simulink model "exp3"  (R2019a)
settings: Solver=FixedStepAuto  StartTime=0.0  StopTime=1e-1  FixedStep=1e-7  RelTol=1e-3
libraries: dsparch4 x1, simulink x1
settings Model: Creator=marco  LastModifiedBy=marco

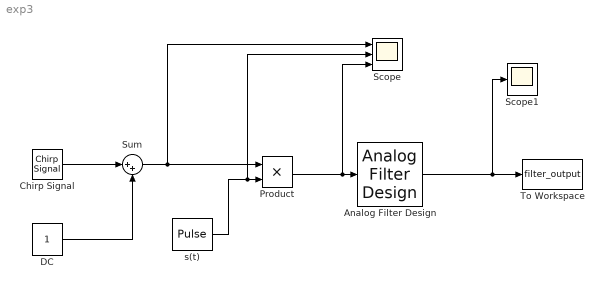
== system exp3 ==
  Analog Filter Design : dsparch4/Analog Filter Design  method=Butterworth  filttype=Bandpass  N=3  Wlo=2*pi*980e3  Whi=2*pi*1020e3  Rp=2  Rs=40
  Chirp Signal : simulink/Sources/Chirp Signal  f1=100  T=0.1  f2=4e3
  DC : Constant
  Product : Product
  Scope : Scope  NumInputPorts=3
  Scope1 : Scope
  Sum : Sum  Inputs=|++
  To Workspace : ToWorkspace  VariableName=filter_output  SaveFormat=Timeseries  SampleTime=1e-7
  "s(t) " : DiscretePulseGenerator  PulseType=Time based  Period=1e-6  PulseWidth=50
  wires:
  Product/1 -> Scope/3, Analog Filter Design/1
  Sum/1 -> Scope/1, Product/1
  Chirp Signal/1 -> Sum/1
  DC/1 -> Sum/2
  "s(t) "/1 -> Scope/2, Product/2
  Analog Filter Design/1 -> Scope1/1, To Workspace/1
